simulink model "GPS_pll_148"  (Simulink 6.1)
settings: Solver=ode45  StartTime=0.0  StopTime=2  RelTol=1e-5
values from neighbouring files (symbols this model uses):
  Ga = 2    [GPS_pll_init.m]    (also in GPS_pll_init_148.m = 0.0625; GPS_pll_init_bak.m = 0.03125)
  Gb = 2    [GPS_pll_init.m]    (also in GPS_pll_init_148.m = 16; GPS_pll_init_bak.m)
  Gdac = 2^-16*5    (= 7.62939453125e-05)    [GPS_pll_init.m]    (also in GPS_pll_init_148.m; GPS_pll_init_bak.m = 5.03540039062e-05)
  Kv = 4e-6    (= 4e-06)    [GPS_pll_init.m]    (also in GPS_pll_init_148.m = 9e-05; GPS_pll_init_bak.m)
  Ts = 1/100e6    (= 1e-08)    [GPS_pll_init.m]    (also in GPS_pll_init_148.m = 6.73400673401e-09; GPS_pll_init_bak.m = 5e-09)
  Ur = 62500    [GPS_pll_init_148.m]
libraries: simulink x1
settings Model: LastModifiedBy=jkh
settings DataIOCC: SignalLoggingName=sigsOut
settings HardwareCC: TargetUnknown=on

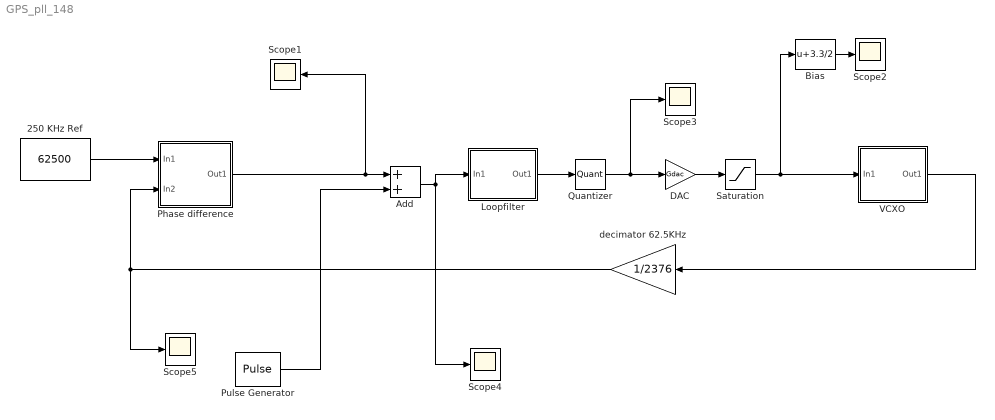
== system GPS_pll_148 ==
  250 KHz Ref : Constant  Value=62500
  Add : Sum  OutScaling=2^-10
  Bias : Bias  Bias=3.3/2
  DAC : Gain  Gain=Gdac  SaturateOnIntegerOverflow=on
  Loopfilter : Subsystem
  Phase difference : Subsystem
  Pulse Generator : DiscretePulseGenerator  PulseType=Time based  Amplitude=1636  Period=1  PulseWidth=50
  Quantizer : Quantizer  QuantizationInterval=1
  Saturation : Saturate  UpperLimit=3.3/2  LowerLimit=-3.3/2
  Scope{1..5} (5 alike) : Scope
      Scope1 settings: TimeRange=0.2  YMin=-8.5  YMax=1.5  SampleInput=on
      Scope2 settings: YMin=1.49  YMax=1.65  SaveName=ScopeData2  SampleInput=on
      Scope3 settings: SaveName=ScopeData3  SampleInput=on
      Scope4 settings: TimeRange=1  YMin=0  YMax=300  SaveName=ScopeData8  SampleInput=on
      Scope5 settings: TimeRange=1  YMin=62494  YMax=62506  SampleInput=on
  VCXO : Subsystem
  decimator 62.5KHz : Gain  Orientation=left  Gain=1/2376  SaturateOnIntegerOverflow=on
  wires:
  250 KHz Ref/1 -> Phase difference/1(In1)
  VCXO/1(Out1) -> decimator 62.5KHz/1
  Phase difference/1(Out1) -> Add/1, Scope1/1
  DAC/1 -> Saturation/1
  Quantizer/1 -> DAC/1, Scope3/1
  Saturation/1 -> Bias/1, VCXO/1(In1)
  Loopfilter/1(Out1) -> Quantizer/1
  Add/1 -> Loopfilter/1(In1), Scope4/1
  Bias/1 -> Scope2/1
  Pulse Generator/1 -> Add/2
  decimator 62.5KHz/1 -> Phase difference/2(In2), Scope5/1

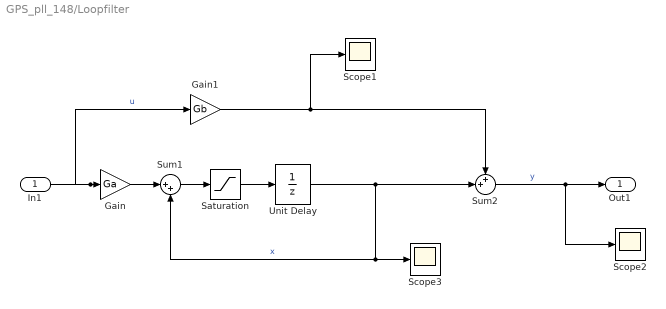
== system GPS_pll_148/Loopfilter ==
  In1 : Inport  Port=1  LatchInput=off
  Gain : Gain  Gain=Ga  SaturateOnIntegerOverflow=on
  Gain1 : Gain  Gain=Gb  SaturateOnIntegerOverflow=on
  Saturation : Saturate  UpperLimit=2^15*(3.3/5)  LowerLimit=-2^15*(3.3/5)
  Scope1 : Scope
      settings: SaveName=ScopeData7  SampleInput=on
  Scope2 : Scope
      settings: YMin=21500  YMax=31500  SaveName=ScopeData9  SampleInput=on
  Scope3 : Scope
      settings: YMin=21626.9  YMax=21626.9  SaveName=ScopeData4  SampleInput=on
  Sum1 : Sum  Inputs=|++  SaturateOnIntegerOverflow=on
  Sum2 : Sum  Inputs=++|  SaturateOnIntegerOverflow=on
  Unit Delay : UnitDelay  SampleTime=1/Ur
  Out1 : Outport
  wires:
  Gain1/1 -> Sum2/1, Scope1/1
  Sum2/1 -> Out1/1, Scope2/1  "y"
  Gain/1 -> Sum1/1
  Sum1/1 -> Saturation/1
  Saturation/1 -> Unit Delay/1
  Unit Delay/1 -> Sum2/2, Sum1/2, Scope3/1  "x"
  In1/1 -> Gain1/1, Gain/1  "u"

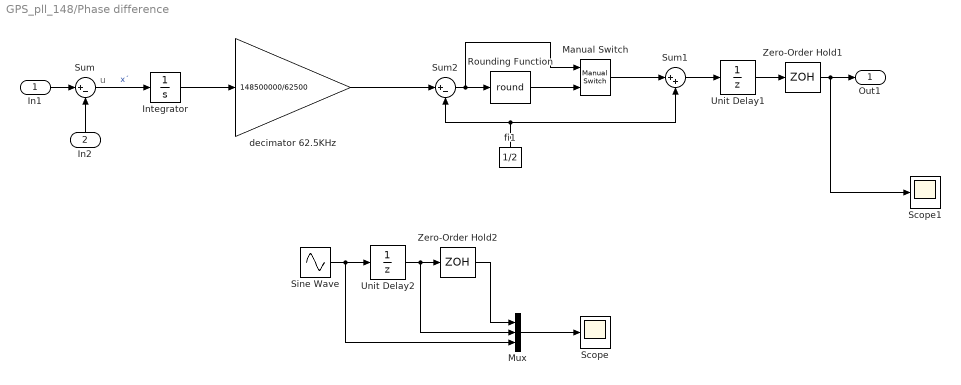
== system GPS_pll_148/Phase difference ==
  note: u
  In1 : Inport  Port=1  LatchInput=off
  In2 : Inport  Orientation=up  Port=2  LatchInput=off
  Integrator : Integrator
  Manual Switch : simulink/Signal Routing/Manual Switch  sw=0  action=0
  Mux : Mux  Inputs=3
  Rounding Function : Rounding  Operator=round
  Scope : Scope
      settings: SaveName=ScopeData6  SampleInput=on
  Scope1 : Scope
      settings: YMin=10800  YMax=11900  SaveName=ScopeData5  SampleInput=on
  Sine Wave : Sin  SampleTime=0
  Sum : Sum  Inputs=|+-  SaturateOnIntegerOverflow=on
  Sum1 : Sum  Inputs=|++  SaturateOnIntegerOverflow=on
  Sum2 : Sum  Inputs=|+-  SaturateOnIntegerOverflow=on
  Unit Delay1 : UnitDelay  SampleTime=0.5*1/Ur
  Unit Delay2 : UnitDelay  SampleTime=0.5
  Zero-Order Hold1 : ZeroOrderHold  SampleTime=1/Ur
  Zero-Order Hold2 : ZeroOrderHold
  decimator 62.5KHz : Gain  Gain=148500000/62500  SaturateOnIntegerOverflow=on
  fi1 : Constant  Orientation=up  Value=1/2
  Out1 : Outport
  wires:
  Sum/1 -> Integrator/1  "x´"
  In2/1 -> Sum/2
  Integrator/1 -> decimator 62.5KHz/1
  In1/1 -> Sum/1
  fi1/1 -> Sum1/2, Sum2/2
  Sum2/1 -> Manual Switch/1, Rounding Function/1
  Manual Switch/1 -> Sum1/1
  Rounding Function/1 -> Manual Switch/2
  Zero-Order Hold1/1 -> Out1/1, Scope1/1
  Unit Delay2/1 -> Zero-Order Hold2/1, Mux/2
  Sine Wave/1 -> Unit Delay2/1, Mux/3
  Zero-Order Hold2/1 -> Mux/1
  Mux/1 -> Scope/1
  decimator 62.5KHz/1 -> Sum2/1
  Sum1/1 -> Unit Delay1/1
  Unit Delay1/1 -> Zero-Order Hold1/1

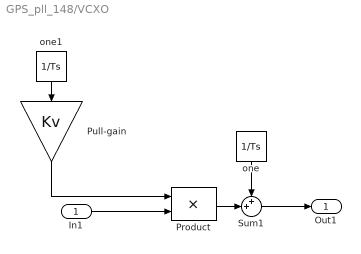
== system GPS_pll_148/VCXO ==
  In1 : Inport  Port=1  LatchInput=off
  Product : Product  SaturateOnIntegerOverflow=on
  "Pull-gain " : Gain  Orientation=down  Gain=Kv  SaturateOnIntegerOverflow=on
  Sum1 : Sum  Inputs=++|  SaturateOnIntegerOverflow=on
  one : Constant  Orientation=down  Value=1/Ts
  one1 : Constant  Orientation=down  Value=1/Ts
  Out1 : Outport
  wires:
  one1/1 -> "Pull-gain "/1
  Product/1 -> Sum1/2
  one/1 -> Sum1/1
  Sum1/1 -> Out1/1
  In1/1 -> Product/2
  "Pull-gain "/1 -> Product/1
